simulink library "Chassis_1Axle"  (R2020a)
settings: Solver=VariableStepAuto  StartTime=0.0  StopTime=10.0  RelTol=1e-3
undefined symbols (not defined in the file): Init, Vehicle
libraries: sm_car_lib x3, Tire_Models x2, Aero_Coefficients x1, Body x1
Description:
  | Copyright 2020 The MathWorks, Inc.
settings Model: Creator=smiller  LastModifiedBy=smiller
settings DataIOCC: ReturnWorkspaceOutputs=off
settings DebuggingCC: ArithmeticOperatorsInVariantConditions=warning
settings SFSimCC: CustomCodeUndefinedFunction=UseInterfaceOnly

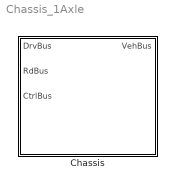
== system Chassis_1Axle ==
  Chassis : Subsystem  Tag=PublishSubsystem  VariantControl=Chassis  mask(Chassis){Chassis=Vehicle.Chassis, Init=Init, InitTriggerDropdown=1}
      mask prompts: Chassis "Vehicle Parameters"; Init "Initial Values"; InitTriggerDropdown "Initialization Trigger Dropdown"
      mask help: Models vehicle chassis, with suspension, body, tires, springs, and dampers.
      mask init:
      | curblk = gcb;
      | 
      | % Trigger Mask Initialization for 
      | % variant subsystems below this level
      | sm_car_lib_maskInitTrigger(curblk)
      mask Help: web('sm_car_doc_chassis.html')
      mask TypeOptions InitTriggerDropdown: 0 | 1

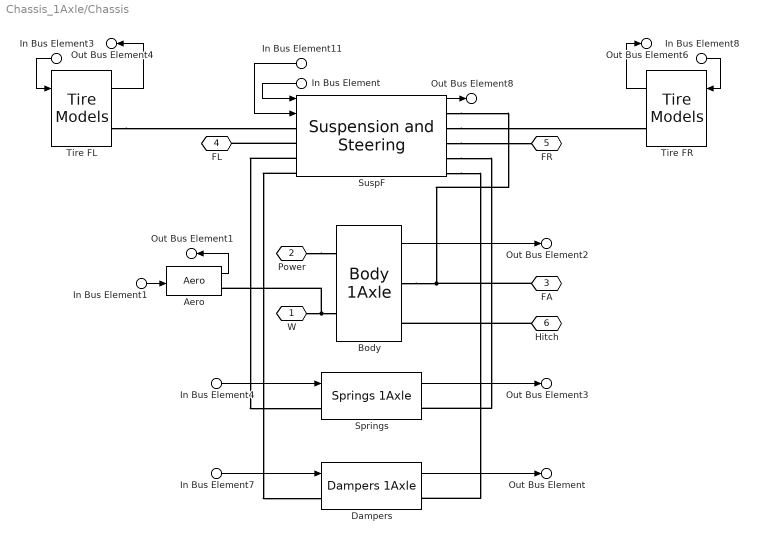
== system Chassis_1Axle/Chassis ==
  In Bus Element11 : Inport  PortName=DrvBus
  In Bus Element3 : Inport  Port=2  PortName=RdBus  Element=FL
  In Bus Element8 : Inport  Port=2  PortName=RdBus  Element=FR
  In Bus Element1 : Inport  Port=2  PortName=RdBus  Element=fWindTrailer
  In Bus Element7 : Inport  Port=3  PortName=CtrlBus  Element=Damper
  In Bus Element : Inport  Port=3  PortName=CtrlBus  Element=SuspF
  In Bus Element4 : Inport  Port=3  PortName=CtrlBus  Element=Spring
  Aero : Aero_Coefficients/Aero  CL=Chassis.Aero.CL.Value  CD=Chassis.Aero.CD.Value  rho=Chassis.Aero.rho_air.Value  A=Chassis.Aero.ARef.Value  sCentreOfPressure=Chassis.Aero.sPressureCentre.Value  clr_hp=Visual.hp.clr  opc_hp=Visual.hp.opc  rad_hp=Visual.hp.rad
  Body : Body/Body 1Axle  hp_mount_fa=Chassis.Body.sAxleF.Value  hp_mount_hitch=Chassis.Body.sHitch.Value  hp_mount_power=Chassis.Body.sPower.Value  hp_chassis_cg=Chassis.Body.sCG.Value  chassis_mass=Chassis.Body.m.Value  chassis_inertia=Chassis.Body.J.Value  clr_chassis_hp_cg=Visual.hp.clr  opc_chassis_hp_cg=Visual.hp.opc  size_chassis_hp_cg=Visual.hp.rad  BodyGeometry=Chassis.Body.BodyGeometry  InitTriggerDropdown=1
  Dampers : sm_car_lib/Springs Dampers/Dampers 1Axle  VariantControl=Variant1  LabelModeActiveChoice=Independent  Damper=Vehicle.Chassis.Damper  VariantLabel=Vehicle.Chassis.Damper.class.Value  InitTriggerDropdown=1
      settings: AttributesFormatString=%<ActiveVariant>
  Springs : sm_car_lib/Springs Dampers/Springs 1Axle  VariantControl=Variant1  LabelModeActiveChoice=Independent  Spring=Vehicle.Chassis.Spring  VariantLabel=Vehicle.Chassis.Spring.class.Value  InitTriggerDropdown=1
      settings: AttributesFormatString=%<ActiveVariant>
  SuspF : sm_car_lib/Suspensions/Suspension and Steering  VariantControl=Variant1  LabelModeActiveChoice=Linkage  Susp=Chassis.SuspF  Init=Init.Front  VariantLabel=Chassis.SuspF.class.Value  InitTriggerDropdown=1
      settings: AttributesFormatString=%<LabelModeActiveChoice>
  Tire FL : Tire_Models/Tire Models  Tag=PublishSubsystem  VariantControl=Variant1  LabelModeActiveChoice=MFEval  popup_leftRight=Left  tir_index=21  Tire=Chassis.TireF  VariantLabel=Chassis.TireF.class.Value  InitTriggerDropdown=1
      settings: AttributesFormatString=%<ActiveVariant>
  Tire FR : Tire_Models/Tire Models  Tag=PublishSubsystem  VariantControl=Variant1  LabelModeActiveChoice=MFEval  popup_leftRight=Right  tir_index=22  Tire=Chassis.TireF  VariantLabel=Chassis.TireF.class.Value  InitTriggerDropdown=1
      settings: AttributesFormatString=%<ActiveVariant>
  W : PMIOPort  Side=Right
  Power : PMIOPort  Port=2  Side=Right
  FA : PMIOPort  Port=3  Side=Left
  FL : PMIOPort  Port=4  Side=Left
  FR : PMIOPort  Port=5  Side=Right
  Hitch : PMIOPort  Port=6  Side=Right
  Out Bus Element4 : Outport  VectorParamsAs1DForOutWhenUnconnected=off  PortName=VehBus  Element=WhlFL
  Out Bus Element6 : Outport  VectorParamsAs1DForOutWhenUnconnected=off  PortName=VehBus  Element=WhlFR
  Out Bus Element1 : Outport  VectorParamsAs1DForOutWhenUnconnected=off  PortName=VehBus  Element=Aero
  Out Bus Element : Outport  VectorParamsAs1DForOutWhenUnconnected=off  PortName=VehBus  Element=Damper
  Out Bus Element3 : Outport  VectorParamsAs1DForOutWhenUnconnected=off  PortName=VehBus  Element=Spring
  Out Bus Element8 : Outport  VectorParamsAs1DForOutWhenUnconnected=off  PortName=VehBus  Element=SuspF
  Out Bus Element2 : Outport  VectorParamsAs1DForOutWhenUnconnected=off  PortName=VehBus  Element=Body
  wires:
  Springs/1 -> Out Bus Element3/1
  Dampers/1 -> Out Bus Element/1
  In Bus Element3/1 -> Tire FL/1
  Tire FR/1 -> Out Bus Element6/1
  In Bus Element8/1 -> Tire FR/1
  Tire FL/1 -> Out Bus Element4/1
  In Bus Element11/1 -> SuspF/2
  SuspF/1 -> Out Bus Element8/1
  In Bus Element/1 -> SuspF/1
  In Bus Element7/1 -> Dampers/1
  In Bus Element4/1 -> Springs/1
  Aero/1 -> Out Bus Element1/1
  In Bus Element1/1 -> Aero/1
  Body/1 -> Out Bus Element2/1
  connections:
  W/RConn1 -- Aero/RConn1 -- Body/LConn2
  SuspF/LConn2 -- FL/RConn1
  SuspF/RConn3 -- FR/RConn1
  SuspF/RConn2 -- Tire FR/RConn1
  Tire FL/RConn1 -- SuspF/LConn1
  FA/RConn1 -- Body/RConn1 -- SuspF/RConn1
  SuspF/LConn3 -- Springs/LConn1
  SuspF/RConn4 -- Springs/RConn1
  SuspF/LConn4 -- Dampers/LConn1
  SuspF/RConn5 -- Dampers/RConn1
  Hitch/RConn1 -- Body/RConn2
  Power/RConn1 -- Body/LConn1
